simulink model "LFSR_1_2"  (R2020b)
settings: Solver=VariableStepAuto  StartTime=0.0  StopTime=10.0  RelTol=1e-3
settings Model: Creator=caeuser  LastModifiedBy=caeuser

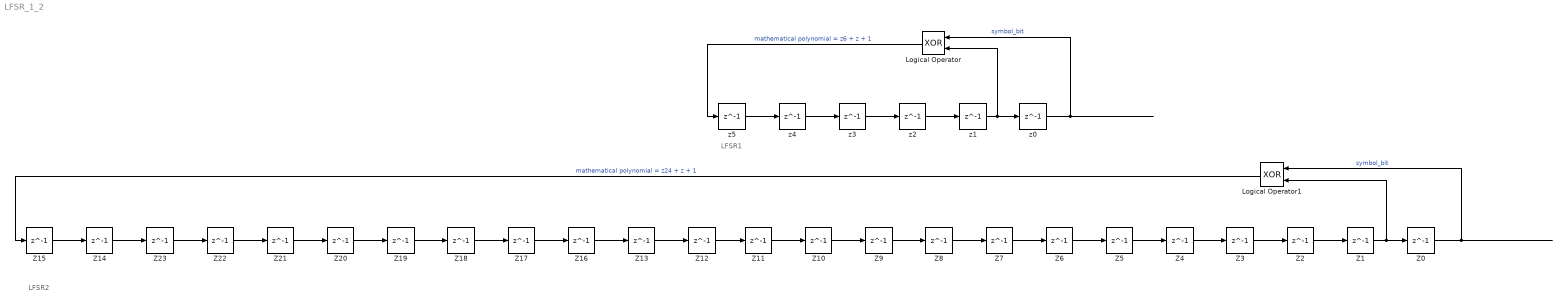
== system LFSR_1_2 ==
  note: LFSR2
  note: LFSR1
  Logical Operator : Logic  Operator=XOR  AllPortsSameDT=off  OutDataTypeStr=boolean
  Logical Operator1 : Logic  Operator=XOR  AllPortsSameDT=off  OutDataTypeStr=boolean
  Z{0..23} (24 alike) : Delay  DelayLength=1
  z{0..5} (6 alike) : Delay  DelayLength=1
  wires:
  z1/1 -> Logical Operator/2, z0/1
  z2/1 -> z1/1
  z3/1 -> z2/1
  z4/1 -> z3/1
  Logical Operator/1 -> z5/1  "mathematical polynomial = z6 + z + 1"
  z5/1 -> z4/1
  z0/1 -> Logical Operator/1  "symbol_bit"
  Z15/1 -> Z14/1
  Z14/1 -> Z23/1
  Z23/1 -> Z22/1
  Z22/1 -> Z21/1
  Z21/1 -> Z20/1
  Z20/1 -> Z19/1
  Z19/1 -> Z18/1
  Z18/1 -> Z17/1
  Z17/1 -> Z16/1
  Z16/1 -> Z13/1
  Z13/1 -> Z12/1
  Z12/1 -> Z11/1
  Z11/1 -> Z10/1
  Z10/1 -> Z9/1
  Z9/1 -> Z8/1
  Z8/1 -> Z7/1
  Z7/1 -> Z6/1
  Z6/1 -> Z5/1
  Z5/1 -> Z4/1
  Z4/1 -> Z3/1
  Z3/1 -> Z2/1
  Z2/1 -> Z1/1
  Z1/1 -> Logical Operator1/2, Z0/1
  Z0/1 -> Logical Operator1/1  "symbol_bit"
  Logical Operator1/1 -> Z15/1  "mathematical polynomial = z24 + z + 1"
